simulink library "cdh_bus"  (R2018b)
settings: Solver=VariableStepAuto  StartTime=0.0  StopTime=10.0  RelTol=1e-3
undefined symbols (not defined in the file): fswParams
libraries: clock_lib x1
settings Model: Creator=colem  LastModifiedBy=colem

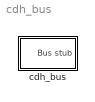
== system cdh_bus ==
  cdh_bus : Subsystem

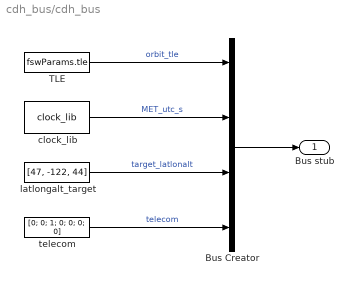
== system cdh_bus/cdh_bus ==
  Bus Creator : BusCreator  Inputs=4
  TLE : Constant  Value=fswParams.tle  SampleTime=fswParams.sample_time_s
  clock_lib : clock_lib/clock_lib  SystemSampleTime=-1
  latlongalt_target : Constant  Value=[47, -122, 44]  SampleTime=fswParams.sample_time_s
  telecom : Constant  Value=[0; 0; 1; 0; 0; 0; 0]  SampleTime=fswParams.sample_time_s
  Bus stub : Outport
  wires:
  Bus Creator/1 -> Bus stub/1
  telecom/1 -> Bus Creator/4  "telecom"
  latlongalt_target/1 -> Bus Creator/3  "target_latlonalt"
  clock_lib/1 -> Bus Creator/2  "MET_utc_s"
  TLE/1 -> Bus Creator/1  "orbit_tle"
